simulink model "power_KundurTwoAreaSystem"  (R2021b)
settings: Solver=VariableStepAuto  StartTime=0.0  StopTime=20  MaxStep=1/60  RelTol=1e-4
PreLoadFcn:
  | Ts=50e-6;
  | Tctrl=2*Ts;
  | PSSMODEL=1;
model workspace (MAT data in the model file):
  LOL = 0
undefined symbols (not defined in the file or in its folder): D1, Delta
libraries: spsGenericPowerSystemStabilizerLib x8, spsThreePhaseVIMeasurementLib x6, spsLoadFlowBusLib x6, spsThreePhaseParallelRLCLoadLib x4, spsThreePhasePISectionLineLib x4, spsSynchronousMachinepuStandardLib x4, spsExcitationSystemLib x4, spsSteamTurbineandGovernorLib x4, spsThreePhaseSeriesRLCLoadLib x4, spsThreePhaseTransformerTwoWindingsLib x4, spsThreePhaseBreakerLib x2, spsDistributedParametersLineLib x2
(part 1 of 2)
settings Model: ARTEMISmethode_block_infos=$$__separator__$$  Creator=The MathWorks, Inc.  LastModifiedBy=Pavel
settings SolverCC: AlgebraicLoopSolver=TrustRegion
settings DataIOCC: SaveOutput=off  SignalLogging=off  DSMLogging=off  SaveTime=off  ReturnWorkspaceOutputs=off  TimeSaveName=t  SignalLoggingName=sigsOut
settings OptimizationCC: BlockReduction=off  BooleanDataType=off  OptimizeBlockIOStorage=off  BufferReuse=off  GlobalBufferReuse=off  ExpressionFolding=off  ExpressionDepthLimit=2147483647  LocalBlockOutputs=off  InitFltsAndDblsToZero=on  LifeSpan=inf  OptimizeDataStoreBuffers=off  BusAssignmentInplaceUpdate=off
settings DebuggingCC: SaveWithParameterizedLinksMsg=none  SignalResolutionControl=TryResolveAllWithWarning  MultiTaskDSMMsg=warning  MultiTaskCondExecSysMsg=none  FcnCallInpInsideContextMsg=warning  UnconnectedOutputMsg=none  StateNameClashWarn=warning  SFUnexpectedBacktrackingDiag=warning  SFNoUnconditionalDefaultTransitionDiag=warning  SFExecutionAtInitializationDiag=none  SFMachineParentedDataDiag=warning  ArithmeticOperatorsInVariantConditions=warning
settings HardwareCC: ProdBitPerPointer=32  ProdBitPerSizeT=32  ProdBitPerPtrDiffT=32  ProdLargestAtomicFloat=None  ProdIntDivRoundTo=Undefined  ProdEndianess=Unspecified  ProdWordSize=32  ProdHWDeviceType=32-bit Generic  TargetBitPerPointer=64  TargetBitPerSizeT=64  TargetBitPerPtrDiffT=64  TargetLongLongMode=on  TargetIntDivRoundTo=Zero  TargetEndianess=LittleEndian  TargetWordSize=64  TargetHWDeviceType=MATLAB Host  ProdEqTarget=off
settings ModelReferenceCC: PropagateSignalLabelsOutOfModel=off
settings SFSimCC: SimUseLocalCustomCode=off  CustomCodeUndefinedFunction=UseInterfaceOnly
settings RTWCC: RTWUseLocalCustomCode=off
settings CodeAppCC: StateflowObjectComments=on
settings GRTTargetCC: TargetFcnLib=ansi_tfl_tmw.mat  TargetLangStandard=C89/C90 (ANSI)  CombineOutputUpdateFcns=off  GRTInterface=on
settings ConfigComp: CovMetricSettings=dw  CovSaveCumulativeToWorkspaceVar=on  CovSaveSingleToWorkspaceVar=on  CovExternalEMLEnable=off  CovSFcnEnable=off
settings SimscapeCC: SimscapeNormalizeSystem=off  SimscapeNominalValues={1, 'bar'; 1, 'cm^3/s'; 1, 'bar*kg/s'; 1, 'kJ/kg'; 1, 'kW'; }

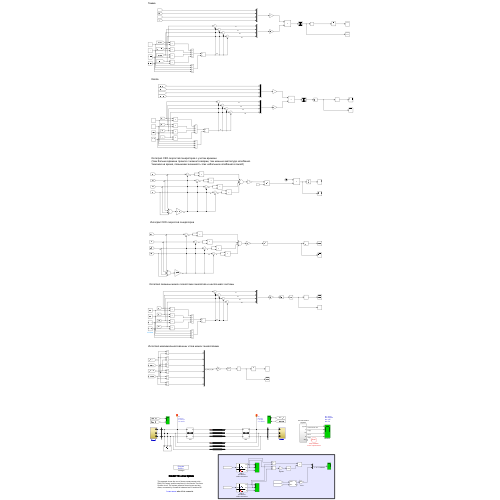
[thumbnail: Simulink's stored preview of the top-level diagram]
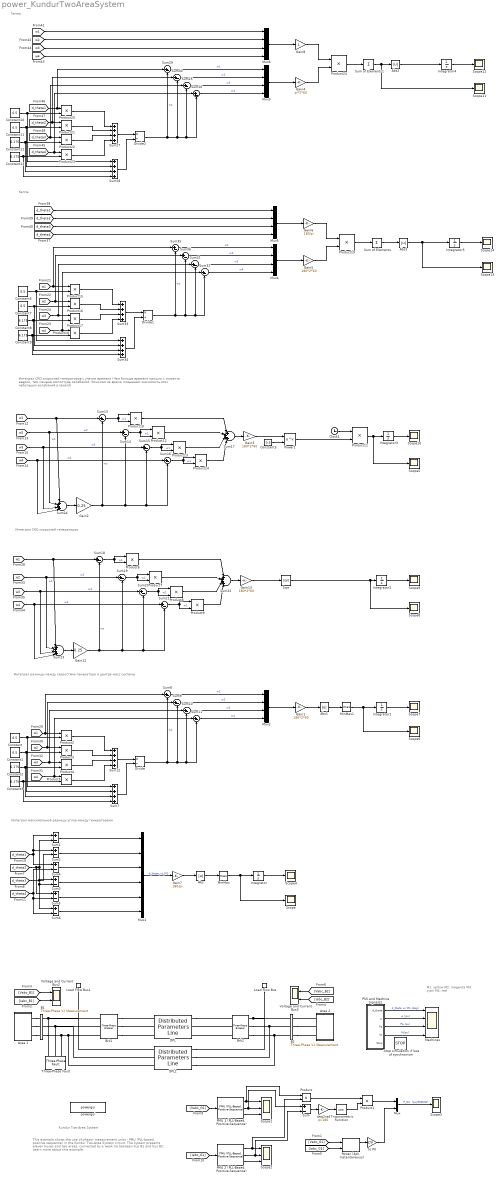
== system power_KundurTwoAreaSystem ==
  note: Интеграл максимальной разницы углов между генераторами
  note: This example shows the use of phasor measurement units - PMU (PLL-based, positive sequence) in the Kundur Two-Area System circuit. The system presents eleven buses and two areas, connected by a weak tie between bus B1 and bus B2.
      |
      | Learn more about this example.
  note: M1: yellow
      | M2: magenta
      | M3: cyan
      | M4: red
  note: Kundur Two-Area System
  note: Интеграл разницы между скоростями генератора и центра масс системы
  note: Интеграл СКО скоростей генераторов
  note: Интеграл СКО скоростей генераторов с учетом времени
      | (Чем больше времени прошло с момента аварии, тем меньше амплитуда колебаний. Умножая на время, повышаем значимость этих небольших колебаний в reward)
  note: Каппа
  note: Гамма
  " Brk2" : spsThreePhaseBreakerLib/Three-Phase Breaker  InitialState=closed  SwitchA=on  SwitchB=on  SwitchC=on  SwitchTimes=[2+12]*100  External=off  BreakerResistance=0.001  SnubberResistance=1e6  SnubberCapacitance=0  Measurements=None
      settings: AttributesFormatString=\n
  Abs{,1..3} (4 alike) : Abs  SaturateOnIntegerOverflow=on
  Area 1 : Subsystem
  Area 2 : Subsystem
  B1 : spsThreePhaseVIMeasurementLib/Three-Phase V-I Measurement  VoltageMeasurement=phase-to-ground  SetLabelV=on  LabelV=Vabc_B1  Vpu=on  VpuLL=off  CurrentMeasurement=yes  SetLabelI=on  LabelI=Iabc_B1  Ipu=off  Pbase=100e6  Vbase=230e3  OutputType=Complex  PhasorSimulation=off  PSBequivalent=0
  B2 : spsThreePhaseVIMeasurementLib/Three-Phase V-I Measurement  VoltageMeasurement=phase-to-ground  SetLabelV=on  LabelV=Vabc_B2  Vpu=off  VpuLL=off  CurrentMeasurement=yes  SetLabelI=on  LabelI=Iabc_B2  Ipu=off  Pbase=100e6  Vbase=500e3  OutputType=Complex  PhasorSimulation=off  PSBequivalent=0
  Brk1 : spsThreePhaseBreakerLib/Three-Phase Breaker  InitialState=closed  SwitchA=off  SwitchB=off  SwitchC=off  SwitchTimes=[2+12]  External=off  BreakerResistance=0.001  SnubberResistance=inf  SnubberCapacitance=0  Measurements=None
      settings: AttributesFormatString=\n
  Clock1 : Clock
  Constant{,1,6..7,10..11} (6 alike) : Constant  Value=6.5
  Constant{2..3,8..9,12..13} (6 alike) : Constant  Value=6.175
  Constant5 : Constant  Value=0.5
  DPL : spsDistributedParametersLineLib/Distributed Parameters Line  Phases=3  Length=220  Frequency=60  Resistance=[0.0001*529 1.61]  Inductance=[0.001*529/(377) 0.0061]  Capacitance=[0.00175/529/(377) 5.2489e-9]  x1=[-0.00125 4.24168847071057e-05 242154.913453712 -378268.611075755;-0.0012 3.78652229655789e-05 249241.699355128 -373637.156528352;-0.00115 3.33001078906322e-05 256239.930867557 -368872.950478352;-0.0011 2.87231614459144e-05 263147.121552666 -363977.68562548;-0.00105 2.41360097987035e-05 269960.817318493 -358953.101234027;-0.001 1.95402827421377e-05 276678.597291377 -353800.982514903;-0.00095 1.49376131161569e-05 283298.074676081 -348523.159991357;-0.0009 1.03296362273631e-05 289816.897603809 -343121.5088486;-0.00085 5.71798926800358e-06 296232.749967817 -337597.948267562;-0.0008 1.10431073428398e-06 302543.352246308 -331954.440743018;-0.00075 -3.50976015578118e-06 308746.462312342 -326192.991386318;-0.0007 -8.12258404477517e-06 314839.876230449 -320315.647212985;-0.00065 -1.27325220183347e-05 320821.429039679 -314324.496415418;-0.0006 -1.73379361874485e-05 326688.9955228 -308221.667620967;-0.00055 -2.19371902703915e-05 332440.49096138 -302009.329135645;-0.0005 -2.6528650174088e-05 338073.871876476 -295689.688173734;-0.00045 -3.11106845746969e-05 343587.136754673 -289264.990073576;-0.0004 -3.56816654972136e-05 348978.326759211 -282737.517499814;-0.00035 -4.02399688938816e-05 354245.526425954 -276109.589632373;-0.0003 -4.4783975221209e-05 359386.86434394 -269383.561342464;-0.00025 -4.93120700153845e-05 364400.513820286 -262561.822355911;-0.0002 -5.38226444658888e-05 369284.693529209 -255646.796404095;-0.00015 -5.83140959870971e-05 374037.668144913 -248640.940362808;-0.0001 -6.27848287876708e-05 378657.74895815 -241546.743379344;-5e-05 -6.72332544375335e-05 383143.294476206 -234366.72598811]  x2=[-0.00125 0.000104496170581926 -84178.9423133657 -331460.289661515;-0.0012 0.000103951893551609 -77916.4724740299 -332988.025993747;-0.00115 0.000103370682908492 -71626.3192830326 -334397.453265906;-0.0011 0.00010275274515395 -65310.7176018511 -335688.070715193;-0.00105 0.000102098299838323 -58971.9113336904 -336859.419791372;-0.001 0.000101407579482918 -52612.1526262346 -337911.084319696;-0.00095 0.000100680829497386 -46233.7010714696 -338842.690648764;-0.0009 9.9918308092537e-05 -39838.8229028612 -339653.907783284;-0.00085 9.91202861885959e-05 -33429.7901901726 -340344.447501671;-0.0008 9.8287047318945e-05 -27008.8800322094 -340914.064458451;-0.00075 9.7418887529387e-05 -20578.3737477767 -341362.556271432;-0.0007 9.65161152729613e-05 -14140.5560651377 -341689.763593607;-0.00065 9.5579051300352e-05 -7697.71431026073 -341895.570169774;-0.0006 9.46080285459267e-05 -1252.13759414292 -341979.902877835;-0.00055 9.36033920094462e-05 5193.88400049989 -341942.731754782;-0.0005 9.25654986334885e-05 11638.0602328886 -341784.070007336;-0.00045 9.14947171766277e-05 18078.1015178926 -341503.974007263;-0.0004 9.0391428082417e-05 24511.7197395083 -341102.543271336;-0.00035 8.92560233442181e-05 30936.629063816 -340579.920425984;-0.0003 8.80889063659281e-05 37350.5467511257 -339936.291156617;-0.00025 8.6890491818652e-05 43751.1939670238 -339171.884141649;-0.0002 8.5661205493372e-05 50136.2965920319 -338286.970971252;-0.00015 8.44014841496662e-05 56503.5860295907 -337281.866050863;-0.0001 8.31117753605297e-05 62850.8000120818 -336156.926489473;-5e-05 8.1792537353354e-05 69175.6834046 -334912.551972752]  x3=[-0.00125 -1.30073036814727e-07 581.32351976172 1802.01651045561;-0.0012 -1.28650380987693e-07 547.255027379994 1812.65326992482;-0.00115 -1.27182016292879e-07 512.992097892859 1822.64600231838;-0.0011 -1.25668464433268e-07 478.546904756015 1831.99115726607;-0.00105 -1.24110263166629e-07 443.931686182569 1840.68541447882;-0.001 -1.22507966114453e-07 409.158740794855 1848.72568492845;-0.00095 -1.20862142565252e-07 374.240423254795 1856.10911194515;-0.0009 -1.19173377272298e-07 339.189139874342 1862.83307223245;-0.00085 -1.17442270245856e-07 304.017344207581 1868.89517679929;-0.0008 -1.15669436540012e-07 268.737532626037 1874.29327180878;-0.00075 -1.13855506034138e-07 233.362239878777 1879.02543934347;-0.0007 -1.12001123209107e-07 197.904034638869 1883.08999808676;-0.00065 -1.10106946918306e-07 162.375515037798 1886.48550392028;-0.0006 -1.08173650153553e-07 126.789304189405 1889.21075043698;-0.00055 -1.06201919805981e-07 91.1580457049546 1891.26476936975;-0.0005 -1.04192456421996e-07 55.4943992009252 1892.64683093545;-0.00045 -1.02145973954368e-07 19.811035801103 1893.35644409418;-0.0004 -1.00063199508575e-07 -15.8793663654067 1893.39335672376;-0.00035 -9.79448730844584e-08 -51.5641266686583 1892.75755570931;-0.0003 -9.57917473133114e-08 -87.2305664832333 1891.4492669479;-0.00025 -9.36045871904677e-08 -122.866013692895 1889.46895526831;-0.0002 -9.13841698035045e-08 -158.457807192933 1886.81732426584;-0.00015 -8.91312840561466e-08 -193.993301388591 1883.49531605237;-0.0001 -8.68467303879727e-08 -229.459870687988 1879.50411092158;-5e-05 -8.45313204900229e-08 -264.844913987929 1874.84512692967]  x4=[-0.00125 2.86918544594886e-07 -451.193099671548 -3595.35316184637;-0.0012 2.82321210867361e-07 -383.346048401822 -3603.21848238076;-0.00115 2.7762356975792e-07 -315.362796106445 -3609.80359654552;-0.0011 2.72827290316081e-07 -247.26749691125 -3615.10616468092;-0.00105 2.67934076637092e-07 -179.084344751795 -3619.12430280977;-0.001 2.62945667256474e-07 -110.837564777381 -3621.85658330673;-0.00095 2.57863834532326e-07 -42.551404743968 -3623.30203540552;-0.0009 2.52690384015618e-07 25.7498736009369 -3623.46014554392;-0.00085 2.47427153808685e-07 94.0420031383625 -3622.33085754614;-0.0008 2.42076013912157e-07 162.300719999866 -3619.91457264283;-0.00075 2.36638865560559e-07 230.501772188366 -3616.21214932852;-0.0007 2.31117640546812e-07 298.62092819477 -3611.22490305656;-0.00065 2.25514300535872e-07 366.633985607305 -3604.95460577182;-0.0006 2.19830836367765e-07 434.516779710524 -3597.40348528107;-0.00055 2.14069267350247e-07 502.245192070916 -3588.57422446146;-0.0005 2.08231640541355e-07 569.795159106064 -3578.46996030732;-0.00045 2.02320030022099e-07 637.142680634329 -3567.09428281559;-0.0004 1.96336536159546e-07 704.263828401995 -3554.45123371032;-0.00035 1.90283284860576e-07 771.134754584864 -3540.54530500664;-0.0003 1.8416242681655e-07 837.731700261279 -3525.38143741482;-0.00025 1.77976136739188e-07 904.03100385355 -3508.96501858481;-0.0002 1.71726612587897e-07 970.009109534801 -3491.30188119205;-0.00015 1.65416074788851e-07 1035.64257559825 -3472.39830086514;-0.0001 1.59046765446079e-07 1100.90808278592 -3452.26099395617;-5e-05 1.52620947544865e-07 1165.78244257388 -3430.8971151544]  x5=0.00124486354111605  V1=[1.852e-10 2.282e+05 2.282e+05;377 377 377;1.887 0.4815 -1.089]  V2=[4.602e-11 2.307e+05 2.307e+05;377 377 377;0.7797 0.0189 -1.552]  I1=[2.265e-13 336.1 336.1;377 377 377;-2.48 -2.709 2.004]  I2=[2.156e-13 1427 1427;377 377 377;2.209 0.1789 -1.392]  nHarmo=1  Measurements=None  Decoupling=off  VsMag0=0  VrMag0=0  VsAngle0=0  VrAngle0=0  IsMag0=0  IrMag0=0  IsAngle0=0  IrAngle0=0
      settings: SourceProductBaseCode=PS
  DPL2 : spsDistributedParametersLineLib/Distributed Parameters Line  Phases=3  Length=220  Frequency=60  Resistance=[0.0001*529 1.61]  Inductance=[0.001*529/(377) 0.0061]  Capacitance=[0.00175/529/(377) 5.2489e-9]  x1=[-0.00125 4.24158242213737e-05 242154.924794119 -378271.378614112;-0.0012 3.78640919415657e-05 249241.762857399 -373639.923361119;-0.00115 3.32989067301852e-05 256240.046509131 -368875.715622486;-0.0011 2.87218905758001e-05 263147.289292455 -363980.448098539;-0.00105 2.41346696704561e-05 269961.037096901 -358955.860054517;-0.001 1.95388738318982e-05 276678.869030317 -353803.736702629;-0.00095 1.49361359245046e-05 283298.398279006 -348525.908567769;-0.0009 1.03280912791371e-05 289817.272955745 -343124.250837142;-0.00085 5.71637711211663e-06 296233.176935402 -337600.682694019;-0.0008 1.10263194352739e-06 302543.830677843 -331957.16663586;-0.00075 -3.51150498494106e-06 308746.992037843 -326195.707777049;-0.0007 -8.12439429240883e-06 314840.457061706 -320318.353136484;-0.00065 -1.27343970412698e-05 320822.060770326 -314327.190910284;-0.0006 -1.73398753194983e-05 326689.677928386 -308224.349729859;-0.00055 -2.19391928225916e-05 332441.223799449 -302011.997905621;-0.0005 -2.65307154349411e-05 338074.654886655 -295692.342656594;-0.00045 -3.11128118104258e-05 343587.969658762 -289267.629326194;-0.0004 -3.56838539520215e-05 348979.209261284 -282740.140584477;-0.00035 -4.02422177902209e-05 354246.458212461 -276112.195617111;-0.0003 -4.47862837600576e-05 359387.845083821 -269386.149301382;-0.00025 -4.93144373765294e-05 364401.543165091 -262564.391369521;-0.0002 -5.38250698082179e-05 369285.771113215 -255649.345559638;-0.00015 -5.8316578448898e-05 374038.79358526 -248643.468754582;-0.0001 -6.27873674869364e-05 378658.921854975 -241549.250109023;-5e-05 -6.72358484722762e-05 383144.514412783 -234369.210165065]  x2=[-0.00125 0.000104493504401818 -84178.6934931397 -331457.464505496;-0.0012 0.00010394919839188 -77916.2769478754 -332985.196649946;-0.00115 0.00010336795972672 -71626.1771204191 -334394.620739574;-0.0011 0.000102749994917668 -65310.6288532885 -335685.236012713;-0.00105 0.000102095523524678 -58971.8760307105 -336856.583919902;-0.001 0.00010140477807832 -52612.1707813803 -337908.248286806;-0.00095 0.000100678003997161 -46233.7726782906 -338839.855462084;-0.0009 9.99154595005715e-05 -39838.9479359159 -339651.074450143;-0.00085 9.91174155169812e-05 -33429.9686050373 -340341.617028737;-0.0008 9.8284155587617e-05 -27009.1117654942 -340911.237851378;-0.00075 9.74159757657642e-05 -20578.6587171479 -341359.7345345;-0.0007 9.65131845115794e-05 -14140.894169347 -341686.947729366;-0.00065 9.55761025824965e-05 -7698.10542918133 -341892.761178687;-0.0006 9.4605062919263e-05 -1252.58158881211 -341977.101757924;-0.00055 9.36004105276475e-05 5193.3872878313 -341939.93950127;-0.0005 9.25625023558609e-05 11637.5109787003 -341781.287612299;-0.00045 9.14917071677345e-05 18077.4999173319 -341501.202459272;-0.0004 9.03884054117e-05 24511.0660063211 -341099.783555109;-0.00035 8.92529890856178e-05 30935.9234302705 -340577.173522035;-0.0003 8.80858615975021e-05 37349.7894679302 -339933.558040908;-0.00025 8.6887437622192e-05 43750.3853032374 -339169.165785242;-0.0002 8.56581429540196e-05 50135.436834969 -338284.268339967;-0.00015 8.43984143555269e-05 56502.6754847189 -337279.180104931;-0.0001 8.31086994022867e-05 62849.8390029132 -336154.258183199;-5e-05 8.17894563238808e-05 69174.6722725767 -334909.902254172]  x3=[-0.00125 -1.3007666837781e-07 581.370317473745 1802.01238818334;-0.0012 -1.28654069730555e-07 547.301894480357 1812.6500304473;-0.00115 -1.27185760904926e-07 513.039017729903 1822.6436467866;-0.0011 -1.25672263584058e-07 478.593860659345 1831.98968651693;-0.00105 -1.24114115506341e-07 443.978661468976 1840.68482903487;-0.001 -1.22511870274369e-07 409.205718774244 1848.72598499769;-0.00095 -1.20866097158243e-07 374.287387236113 1856.11029742098;-0.0009 -1.19177380893315e-07 339.23607317151 1862.83514269367;-0.00085 -1.17446321472433e-07 304.064230145423 1868.89813151028;-0.0008 -1.15673533932766e-07 268.784354546202 1874.29710971974;-0.00075 -1.13859648137287e-07 233.408981145659 1879.0301590908;-0.0007 -1.1200530855098e-07 197.95067864552 1883.09559799356;-0.00065 -1.10111174011871e-07 162.422045211823 1886.49198199694;-0.0006 -1.08177917496943e-07 126.835703998855 1889.21810438187;-0.00055 -1.06206225883031e-07 91.2042986641984 1891.27299657004;-0.0005 -1.04196799702776e-07 55.5404888765067 1892.65592846806;-0.00045 -1.02150352895732e-07 19.85694581758 1893.36640872679;-0.0004 -1.00067612554704e-07 -15.8336523196446 1893.40418491599;-0.00035 -9.79493186674205e-08 -51.5186248355938 1892.76924361396;-0.0003 -9.57962238536111e-08 -87.185293029451 1891.46181041232;-0.00025 -9.36090930976116e-08 -122.820984703838 1889.48234983585;-0.0002 -9.13887034765653e-08 -158.413038667186 1886.83156517748;-0.00015 -8.91358438843318e-08 -193.948809232198 1883.51039824838;-0.0001 -8.68513147511971e-08 -229.4156707088 1879.52002904333;-5e-05 -8.45359277594841e-08 -264.801021889989 1874.86187532152]  x4=[-0.00125 2.86921266557822e-07 -451.239240117452 -3595.34899258331;-0.0012 2.82323919730767e-07 -383.392259238491 -3603.2151835324;-0.00115 2.77626264559351e-07 -315.409060915391 -3609.80116928392;-0.0011 2.72829970098087e-07 -247.313799254805 -3615.10460986848;-0.00105 2.67936740447559e-07 -179.130668178958 -3619.1236209989;-0.001 2.62948314148962e-07 -110.883892829658 -3621.85677473967;-0.00095 2.57866463566408e-07 -42.5977209612231 -3623.30310001427;-0.0009 2.5269299425721e-07 25.7035856746353 -3623.46208295022;-0.00085 2.4742974433038e-07 93.9957599488946 -3622.33366706165;-0.0008 2.42078583793556e-07 162.254537977216 -3619.91825326933;-0.00075 2.36641413888595e-07 230.455667740787 -3616.2166997583;-0.0007 2.31120166416076e-07 298.574917702953 -3611.23032167288;-0.00065 2.25516803048935e-07 366.588085418558 -3604.96089064947;-0.0006 2.19833314635496e-07 434.471006132967 -3597.41063418706;-0.00055 2.14071720492129e-07 502.199561367681 -3588.58223485583;-0.0005 2.08234067685799e-07 569.749687489525 -3578.478829344;-0.00045 2.02322430306751e-07 637.097384260333 -3567.10400734346;-0.0004 1.96338908731597e-07 704.218723364128 -3554.46181027429;-0.00035 1.90285628877062e-07 771.089856908732 -3540.55672984893;-0.0003 1.84164741444655e-07 837.687025898813 -3525.39370647622;-0.00025 1.77978421156534e-07 903.986568677336 -3508.97812750619;-0.0002 1.71728865982841e-07 969.964929332448 -3491.31582531586;-0.00015 1.65418296360772e-07 1035.59866606677 -3472.41307523712;-0.0001 1.59048954405665e-07 1100.86445952616 -3452.27659332704;-5e-05 1.52623103114388e-07 1165.73912108498 -3430.91353398178]  x5=0.00124486354111605  V1=[5.683e-11 2.282e+05 2.282e+05;377 377 377;0.4068 0.4815 -1.089]  V2=[7.166e-11 2.307e+05 2.307e+05;377 377 377;-0.05108 0.0189 -1.552]  I1=[2.676e-13 336.1 336.1;377 377 377;-1.905 -2.709 2.004]  I2=[9.643e-14 1427 1427;377 377 377;-2.04 0.1789 -1.392]  nHarmo=1  Measurements=None  Decoupling=off  VsMag0=0  VrMag0=0  VsAngle0=0  VrAngle0=0  IsMag0=0  IrMag0=0  IsAngle0=0  IrAngle0=0
      settings: SourceProductBaseCode=PS
  Divide : Product  Inputs=*/
  Divide1 : Product  Inputs=*/
  Divide2 : Product  Inputs=*/
  Gain{1,3,5,13} (4 alike) : Gain  Gain=180*2*60
  Gain12 : Gain  Gain=0.25
  Gain2 : Gain  Gain=0.25
  Gain4 : Gain  Gain=pi*2*60
  Gain6 : Gain  Gain=180/pi
  Gain7 : Gain  Gain=180/pi
  Gain8 : Gain
  Integrator{,1..5} (6 alike) : Integrator
  Load Flow Bus : spsLoadFlowBusLib/Load Flow Bus  LConnTagsString=a  Phases=single  Connectors=on one side  ID=B2  Vbase=230e3  Vref=1  Vangle=0  VLF=1.003  VLFb=1  VLFc=1  angleLF=-11.54  angleLFb=0  angleLFc=0
      settings: AttributesFormatString=%<ID>\n%<Vbase>V\n%<VLF>pu\n%<angleLF>deg.  SourceProductBaseCode=PS
  Load Flow Bus1 : spsLoadFlowBusLib/Load Flow Bus  LConnTagsString=a  Phases=single  Connectors=on one side  ID=B1  Vbase=230e3  Vref=1  Vangle=0  VLF=0.9914  VLFb=1  VLFc=1  angleLF=15.04  angleLFb=0  angleLFc=0
      settings: AttributesFormatString=%<ID>\n%<Vbase>V\n%<VLF>pu\n%<angleLF>deg.  SourceProductBaseCode=PS
  Machines : Scope  NumInputPorts=4
  MinMax : MinMax  Function=max  InputSameDT=on  SaturateOnIntegerOverflow=on
  MinMax1 : MinMax  Function=max  InputSameDT=on  SaturateOnIntegerOverflow=on
  Mux : Mux  Inputs=2
  Mux1 : Mux  Inputs=6
  Mux{2..6} (5 alike) : Mux
  "PMU 1 (PLL-Based, Positive-Sequence)" : spsPMUPLLBasedPositiveSequenceLib/PMU (PLL-Based, Positive-Sequence)  nominalFrequency=60  samplingRate=64  reportingFactor=1
      settings: SourceProductBaseCode=PS
  "PMU 2 (PLL-Based, Positive-Sequence)" : spsPMUPLLBasedPositiveSequenceLib/PMU (PLL-Based, Positive-Sequence)  nominalFrequency=60  samplingRate=64  reportingFactor=1
      settings: SourceProductBaseCode=PS
  PSS and Machine Signals2 : Subsystem
  "Power (3ph, Instantaneous)" : spsPower3phInstantaneousLib/Power (3ph, Instantaneous)
  Power1 : Math  Operator=pow  SaturateOnIntegerOverflow=on
  Product{,1..24} (25 alike) : Product
  Scope{,3..14} (13 alike) : Scope
  Scope1 : Scope  NumInputPorts=3
  Scope2 : Scope  NumInputPorts=3
  Sqrt : Sqrt  SaturateOnIntegerOverflow=on
  Stop simulation if loss of synchronism : Stop
  Sum : Sum  Inputs=+-
  Sum of Elements : Sum  Inputs=+
  Sum of Elements1 : Sum  Inputs=+
  Sum{1..6} (6 alike) : Sum  Inputs=+-  InputSameDT=on  SaturateOnIntegerOverflow=on  OutDataTypeStr=Inherit: Same as first input
  Sum{8..11,13..16,18..21,25..26,29..32,35..36} (20 alike) : Sum  Inputs=|+-
  Sum{7,12,27..28,33..34} (6 alike) : Sum  Inputs=++++  InputSameDT=on  SaturateOnIntegerOverflow=on  OutDataTypeStr=Inherit: Same as first input
  Sum{17,22..24} (4 alike) : Sum  Inputs=|++++|
  Three-Phase Fault : spsThreePhaseFaultLib/Three-Phase Fault  InitialStates=0  FaultA=on  FaultB=on  FaultC=on  GroundFault=on  SwitchTimes=[20 20.25]  External=off  SwitchStatus=NaN  FaultResistance=0.001  GroundResistance=0.001  SnubberResistance=1e6  SnubberCapacitance=inf  Measurements=None
  Trigonometric Function : Trigonometry  Operator=cos
  Voltage and Current Bus2 : Scope  NumInputPorts=2
  Voltage and Current Bus3 : Scope  NumInputPorts=2
  deg2rad : Gain  Gain=pi/180
  powergui : spspowerguiLib/powergui  Priority=2  SimulationMode=Discrete  SampleTime=Ts  frequency=60  Iterations=50  frequencyindice=60  Pbase=100e6  ErrMax=1e-4  UnitsV=kV  UnitsW=MW  buscounter=0  FunctionMessages=off  echomessages=off  EnableUseOfTLC=off  CurrentSourceSwitches=off  DisableSnubberDevices=off  DisableRonSwitches=off  DisableVfSwitches=off  DisplayEquations=off  AutomaticDiscreteSolvers=off  SolverType=Tustin  Interpol=off  ExternalGateDelay=off  methode=off  Ts=0  x0status=blocks  SPID=off  SwTol=0  HookPort=off  NonlinearTolerance=1e-4  nMaxIteration=100  ContinueOnMaxIteration=off  RestoreLinks=warning  ResistiveCurrentMeasurement=off  Frange=logspace(0,3,50)  Ylog=off  Xlog=off  ShowGrid=off  save=off  variable=ZData  structure=0  ZoomFFT=on  StartTime=0.0  cycles=1  DisplayStyle=1  fundamental=60  FreqAxis=off  MaxFrequency=1000  frequencyindicesteady=1  RmsSteady=1  display=off
  to PU : Gain  Gain=2/3
  wires:
  [Iabc_B1] -> Voltage and Current Bus2/2
  [Vabc_B1] -> Voltage and Current Bus2/1
  [Iabc_B2] -> Voltage and Current Bus3/2
  [Vabc_B2] -> Voltage and Current Bus3/1
  PSS and Machine Signals2/1(d_theta) -> Machines/1  "d_theta vs M1 (deg)"
  PSS and Machine Signals2/2(w) -> Machines/2  "w (pu)"
  PSS and Machine Signals2/3(Pa) -> Machines/3  "Pa (pu)"
  PSS and Machine Signals2/4(Vt) -> Machines/4  "Vt(pu)"
  [Iabc_G1] -> "PMU 2 (PLL-Based, Positive-Sequence)"/1
  "PMU 2 (PLL-Based, Positive-Sequence)"/3 -> Scope2/3
  [Vabc_G1] -> "PMU 1 (PLL-Based, Positive-Sequence)"/1
  "PMU 1 (PLL-Based, Positive-Sequence)"/3 -> Scope1/3
  Product/1 -> Product1/1
  [Iabc_G1] -> "Power (3ph, Instantaneous)"/2
  "Power (3ph, Instantaneous)"/1 -> to PU/1
  "PMU 2 (PLL-Based, Positive-Sequence)"/1 -> Product/2, Scope2/1
  [Vabc_G1] -> "Power (3ph, Instantaneous)"/1
  "PMU 2 (PLL-Based, Positive-Sequence)"/2 -> Sum/2, Scope2/2
  deg2rad/1 -> Trigonometric Function/1
  "PMU 1 (PLL-Based, Positive-Sequence)"/1 -> Scope1/1, Product/1
  Trigonometric Function/1 -> Product1/2
  Product1/1 -> Mux/1
  Sum/1 -> deg2rad/1
  to PU/1 -> Mux/2
  "PMU 1 (PLL-Based, Positive-Sequence)"/2 -> Sum/1, Scope1/2
  Mux/1 -> Scope3/1  "P_G1  (pu/900MW)"
  Sum4/1 -> Mux1/3
  Sum2/1 -> Mux1/2
  Sum1/1 -> Mux1/1
  Gain7/1 -> Abs/1
  Abs/1 -> MinMax/1
  Sum5/1 -> Mux1/5
  Sum3/1 -> Mux1/4
  [d_theta1] -> Sum4/1, Sum2/1, Sum1/1
  [d_theta2] -> Sum5/1, Sum1/2, Sum3/1
  [d_theta3] -> Sum6/1, Sum3/2, Sum2/2
  [d_theta4] -> Sum6/2, Sum5/2, Sum4/2
  Mux1/1 -> Gain7/1  "d_theta_vs_M1"
  MinMax/1 -> Integrator/1, Scope/1
  Integrator/1 -> Scope4/1
  Product2/1 -> Sum12/1
  [w1] -> Product2/1, Sum8/1
  [w3] -> Product4/1, Sum10/1
  Sum9/1 -> Mux2/2  "w2"
  Divide/1 -> Sum9/2, Sum10/2, Sum11/2, Sum8/2  "ws"
  [w4] -> Product5/1, Sum11/1
  Sum11/1 -> Mux2/4  "w4"
  Sum8/1 -> Mux2/1  "w1"
  Sum10/1 -> Mux2/3  "w3"
  [w2] -> Product3/1, Sum9/1
  Constant/1 -> Sum7/1, Product2/2
  Constant1/1 -> Sum7/2, Product3/2
  Constant2/1 -> Sum7/3, Product4/2
  Constant3/1 -> Sum7/4, Product5/2
  Product3/1 -> Sum12/2
  Product4/1 -> Sum12/3
  Product5/1 -> Sum12/4
  Sum12/1 -> Divide/1
  Sum7/1 -> Divide/2
  Gain1/1 -> Abs1/1
  Abs1/1 -> MinMax1/1
  MinMax1/1 -> Integrator1/1, Scope6/1
  Integrator1/1 -> Scope7/1
  Mux2/1 -> Gain1/1
  Sqrt/1 -> Scope8/1, Integrator2/1
  Sum23/1 -> Gain12/1
  Product9/1 -> Sum22/4
  Product8/1 -> Sum22/3
  Gain12/1 -> Sum18/2, Sum19/2, Sum20/2, Sum21/2  "ws"
  Product7/1 -> Sum22/2
  Sum21/1 -> Product9/1, Product9/2  "w1"
  Sum22/1 -> Gain13/1
  Sum19/1 -> Product7/1, Product7/2  "w1"
  Product6/1 -> Sum22/1
  [w2] -> Sum23/2, Sum19/1  "w2"
  [w4] -> Sum23/4, Sum21/1  "w4"
  [w1] -> Sum23/1, Sum18/1  "w1"
  Integrator2/1 -> Scope9/1
  Sum18/1 -> Product6/2, Product6/1  "w1"
  Sum20/1 -> Product8/2, Product8/1  "w1"
  [w3] -> Sum23/3, Sum20/1  "w3"
  Gain13/1 -> Sqrt/1
  Integrator3/1 -> Scope10/1
  Clock1/1 -> Product11/1
  Product11/1 -> Scope5/1, Integrator3/1
  Gain3/1 -> Power1/1
  [w3] -> Sum15/1, Sum24/3  "w3"
  Sum15/1 -> Product13/1, Product13/2  "w1"
  Sum13/1 -> Product10/1, Product10/2  "w1"
  [w1] -> Sum13/1, Sum24/1  "w1"
  Constant5/1 -> Power1/2
  [w4] -> Sum16/1, Sum24/4  "w4"
  [w2] -> Sum14/1, Sum24/2  "w2"
  Product10/1 -> Sum17/1
  Sum14/1 -> Product12/2, Product12/1  "w1"
  Sum17/1 -> Gain3/1
  Sum16/1 -> Product14/2, Product14/1  "w1"
  Product12/1 -> Sum17/2
  Gain2/1 -> Sum16/2, Sum15/2, Sum14/2, Sum13/2  "ws"
  Product13/1 -> Sum17/3
  Product14/1 -> Sum17/4
  Sum24/1 -> Gain2/1
  Power1/1 -> Product11/2
  Constant9/1 -> Sum34/4, Product18/2
  Constant6/1 -> Sum34/1, Product15/2
  Sum36/1 -> Mux4/2  "w2"
  [w1] -> Product15/1, Sum35/1
  [w3] -> Product17/1, Sum31/1
  Sum31/1 -> Mux4/3  "w3"
  [w2] -> Product16/1, Sum36/1
  Sum32/1 -> Mux4/4  "w4"
  [w4] -> Product18/1, Sum32/1
  Divide1/1 -> Sum36/2, Sum31/2, Sum32/2, Sum35/2  "ws"
  Product17/1 -> Sum33/3
  Product18/1 -> Sum33/4
  Sum35/1 -> Mux4/1  "w1"
  Sum34/1 -> Divide1/2
  Mux4/1 -> Gain5/1
  Integrator5/1 -> Scope14/1
  Product16/1 -> Sum33/2
  Abs3/1 -> Scope13/1, Integrator5/1
  Constant7/1 -> Sum34/2, Product16/2
  Sum33/1 -> Divide1/1
  Constant8/1 -> Sum34/3, Product17/2
  Product15/1 -> Sum33/1
  [d_theta3] -> Mux5/3
  [d_theta4] -> Mux5/4
  [d_theta2] -> Mux5/2
  [d_theta1] -> Mux5/1
  Mux5/1 -> Gain6/1
  Gain6/1 -> Product19/1
  Gain5/1 -> Product19/2
  Product19/1 -> Sum of Elements/1
  Sum of Elements/1 -> Abs3/1
  Sum of Elements1/1 -> Scope11/1, Abs2/1
  Product24/1 -> Sum of Elements1/1
  Gain4/1 -> Product24/2
  Gain8/1 -> Product24/1
  Mux6/1 -> Gain8/1
  [w1] -> Mux6/1
  [w2] -> Mux6/2
  [w4] -> Mux6/4
  [w3] -> Mux6/3
  Product20/1 -> Sum27/1
  Constant12/1 -> Product22/2, Sum28/3
  Sum27/1 -> Divide2/1
  Constant11/1 -> Product21/2, Sum28/2
  Abs2/1 -> Integrator4/1
  Product21/1 -> Sum27/2
  Integrator4/1 -> Scope12/1
  Mux3/1 -> Gain4/1
  Sum28/1 -> Divide2/2
  Sum29/1 -> Mux3/1  "w1"
  Product23/1 -> Sum27/4
  Product22/1 -> Sum27/3
  Divide2/1 -> Sum29/2, Sum26/2, Sum25/2, Sum30/2  "ws"
  [d_theta4] -> Sum26/1, Product23/1
  Sum26/1 -> Mux3/4  "w4"
  [d_theta2] -> Product21/1, Sum30/1
  Sum25/1 -> Mux3/3  "w3"
  [d_theta3] -> Product22/1, Sum25/1
  [d_theta1] -> Product20/1, Sum29/1
  Sum30/1 -> Mux3/2  "w2"
  Constant10/1 -> Product20/2, Sum28/1
  Constant13/1 -> Product23/2, Sum28/4
  Sum6/1 -> Mux1/6
  connections:
  " Brk2"/RConn1 -- DPL2/RConn1 -- B2/LConn1 -- Load Flow Bus/LConn1
  " Brk2"/RConn2 -- DPL2/RConn2 -- B2/LConn2
  " Brk2"/RConn3 -- DPL2/RConn3 -- B2/LConn3
  B2/RConn3 -- Area 2/LConn3
  B2/RConn2 -- Area 2/LConn2
  Area 2/LConn1 -- B2/RConn1
  Area 1/RConn3 -- B1/LConn3
  Area 1/RConn2 -- B1/LConn2
  Area 1/RConn1 -- B1/LConn1
  " Brk2"/LConn3 -- DPL/RConn3
  " Brk2"/LConn2 -- DPL/RConn2
  DPL/RConn1 -- " Brk2"/LConn1
  Brk1/RConn3 -- DPL/LConn3
  Brk1/RConn2 -- DPL/LConn2
  Brk1/RConn1 -- DPL/LConn1
  DPL2/LConn3 -- B1/RConn3 -- Three-Phase Fault/LConn3 -- Brk1/LConn3
  DPL2/LConn2 -- Brk1/LConn2 -- Three-Phase Fault/LConn2 -- B1/RConn2
  DPL2/LConn1 -- Brk1/LConn1 -- Load Flow Bus1/LConn1 -- Three-Phase Fault/LConn1 -- B1/RConn1

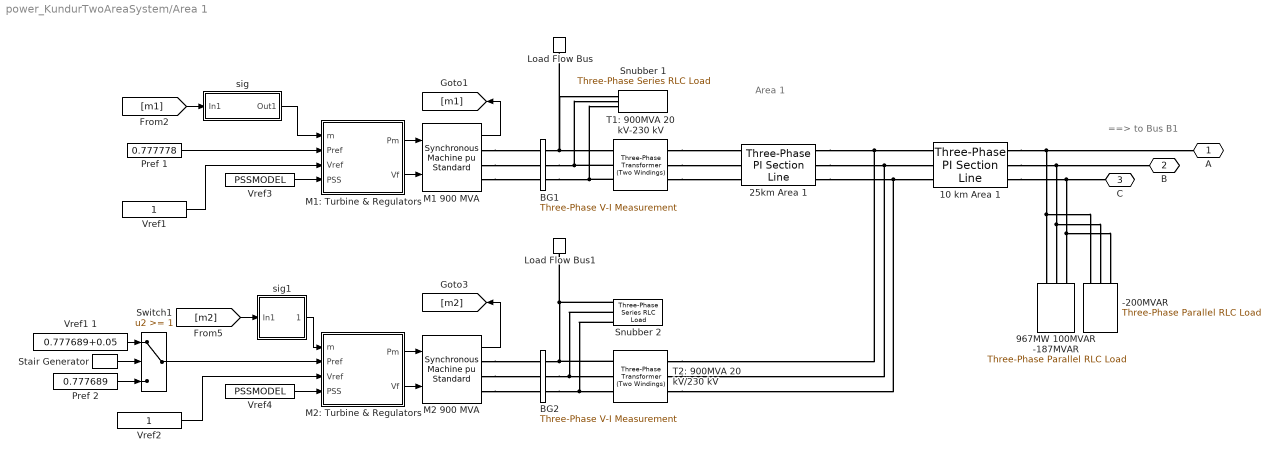
== system power_KundurTwoAreaSystem/Area 1 ==
  note: Area 1
  note: ==> to Bus B1
  -200MVAR : spsThreePhaseParallelRLCLoadLib/Three-Phase Parallel RLC Load  LConnTagsString=A|B|C  Configuration=Y (grounded)  NominalVoltage=230e3  Vabc=[1e3 1e3 1e3]  Vabcp=[1e3 1e3 1e3]  NominalFrequency=60  UnbalancedPower=off  ActivePower=0  InductivePower=0  CapacitivePower=200e6  Pabc=[10e3 9e3 11e3]  QLabc=[100 90 110]  QCabc=[100 90 110]  Pabcp=[10e3 9e3 11e3]  QLabcp=[100 90 110]  QCabcp=[100 90 110]  Measurements=None  LoadType=constant Z
  10 km Area 1 : spsThreePhasePISectionLineLib/Three-Phase PI Section Line  LConnTagsString=a|b|c  RConnTagsString=A|B|C  Length=10  Frequency=60  Resistances=[0.0001*529 1.61]  Inductances=[0.001*529/(377) 0.0061]  Capacitances=[0.00175/529/(377) 5.2489e-9]
  25km Area 1 : spsThreePhasePISectionLineLib/Three-Phase PI Section Line  LConnTagsString=a|b|c  RConnTagsString=A|B|C  Length=25  Frequency=60  Resistances=[0.0001*529 1.61]  Inductances=[0.001*529/(377) 0.0061]  Capacitances=[0.00175/529/(377) 5.2489e-9]
  967MW 100MVAR -187MVAR : spsThreePhaseParallelRLCLoadLib/Three-Phase Parallel RLC Load  LConnTagsString=A|B|C  Configuration=Y (grounded)  NominalVoltage=230e3  Vabc=[1e3 1e3 1e3]  Vabcp=[1e3 1e3 1e3]  NominalFrequency=60  UnbalancedPower=off  ActivePower=167e6  InductivePower=100e6  CapacitivePower=187e6  Pabc=[10e3 9e3 11e3]  QLabc=[100 90 110]  QCabc=[100 90 110]  Pabcp=[10e3 9e3 11e3]  QLabcp=[100 90 110]  QCabcp=[100 90 110]  Measurements=None  LoadType=constant Z
  BG1 : spsThreePhaseVIMeasurementLib/Three-Phase V-I Measurement  VoltageMeasurement=phase-to-ground  SetLabelV=on  LabelV=Vabc_G1  Vpu=on  VpuLL=off  CurrentMeasurement=yes  SetLabelI=on  LabelI=Iabc_G1  Ipu=on  Pbase=900e6  Vbase=20e3  OutputType=Complex  PhasorSimulation=off  PSBequivalent=0
  BG2 : spsThreePhaseVIMeasurementLib/Three-Phase V-I Measurement  VoltageMeasurement=no  SetLabelV=on  LabelV=Vabc_G2  Vpu=on  VpuLL=off  CurrentMeasurement=no  SetLabelI=on  LabelI=Iabc_G2  Ipu=on  Pbase=900e6  Vbase=20e3  OutputType=Complex  PhasorSimulation=off  PSBequivalent=0
  Load Flow Bus : spsLoadFlowBusLib/Load Flow Bus  LConnTagsString=a  Phases=single  Connectors=on one side  ID=M1_Area1  Vbase=20e3  Vref=1  Vangle=0  VLF=1  VLFb=1  VLFc=1  angleLF=10.19  angleLFb=0  angleLFc=0
      settings: AttributesFormatString=%<ID>\n%<Vbase>V\n%<VLF>pu\n%<angleLF>deg.  SourceProductBaseCode=PS
  Load Flow Bus1 : spsLoadFlowBusLib/Load Flow Bus  LConnTagsString=a  Phases=single  Connectors=on one side  ID=M2_Area1  Vbase=20e3  Vref=1  Vangle=0  VLF=1  VLFb=1  VLFc=1  angleLF=0  angleLFb=0  angleLFc=0
      settings: AttributesFormatString=%<ID>\n%<Vbase>V\n%<VLF>pu\n%<angleLF>deg.  SourceProductBaseCode=PS
  M1 900 MVA : spsSynchronousMachinepuStandardLib/Synchronous Machine pu Standard  PresetModel=No  MechanicalLoad=Mechanical power Pm  ShowDetailedParameters=on  RotorType=Round  Units=per unit standard parameters  MeasurementBus=off  NominalParameters="[900E6  20000   60 ]"  Reactances1=[1.8 .3 .25 1.7 .55 .25 .2]  Reactances2=[ 1.305, 0.296, 0.252, 0.474, 0.243, 0.18 ]  dAxisTimeConstants=Open-circuit  qAxisTimeConstants=Open-circuit  TimeConstants1=[]  TimeConstants2=[8 .03 .4 .05]  TimeConstants3=[]  TimeConstants4=[]  TimeConstants5=[ 1.01, 0.053, 0.1 ]  TimeConstants6=[]  TimeConstants7=[]  TimeConstants8=[]  StatorResistance=0.0025  Mechanical="[ 6.5 0  4]"  PolePairs=4  InitialConditions=[0 -31.4247 0.784453 0.784453 0.784453 2.7401 -117.26 122.74 1.83395]  SetSaturation=off  Saturation=[0.6404,0.7127,0.8441,0.9214,0.9956,1.082,1.19,1.316,1.457;0.7,0.7698,0.8872,0.9466,0.9969,1.046,1.1,1.151,1.201]  LoadFlowParameters=[1 700000000 0 0 0]  TsPowergui=0  TsBlock=-1  IterativeModel=Trapezoidal non iterative  IterativeDiscreteModel=Trapezoidal non iterative  BusType=PV  Pref=700000000  Qref=0  Qmin=-inf  Qmax=inf  PLF=0  QLF=0
      settings: SourceProductBaseCode=PS
  M1: Turbine & Regulators : Subsystem
  M2 900 MVA : spsSynchronousMachinepuStandardLib/Synchronous Machine pu Standard  PresetModel=No  MechanicalLoad=Mechanical power Pm  ShowDetailedParameters=on  RotorType=Round  Units=per unit standard parameters  MeasurementBus=off  NominalParameters="[900E6  20000   60 ]"  Reactances1=[1.8 .3 .25 1.7 .55 .25 .2]  Reactances2=[ 1.305, 0.296, 0.252, 0.474, 0.243, 0.18 ]  dAxisTimeConstants=Open-circuit  qAxisTimeConstants=Open-circuit  TimeConstants1=[]  TimeConstants2=[8 .03 .4 .05]  TimeConstants3=[]  TimeConstants4=[]  TimeConstants5=[ 1.01, 0.053, 0.1 ]  TimeConstants6=[]  TimeConstants7=[]  TimeConstants8=[]  StatorResistance=0.0025  Mechanical="[ 6.5 0  4]"  PolePairs=4  InitialConditions=[0 -42.8075 0.788608 0.788608 0.788608 -9.54571 -129.546 110.454 1.86756]  SetSaturation=off  Saturation=[0.6404,0.7127,0.8441,0.9214,0.9956,1.082,1.19,1.316,1.457;0.7,0.7698,0.8872,0.9466,0.9969,1.046,1.1,1.151,1.201]  LoadFlowParameters=[2 700000000 0 0 0]  TsPowergui=0  TsBlock=-1  IterativeModel=Trapezoidal non iterative  IterativeDiscreteModel=Trapezoidal non iterative  BusType=swing  Pref=0  Qref=0  Qmin=-inf  Qmax=inf  PLF=0  QLF=0
      settings: SourceProductBaseCode=PS
  M2: Turbine & Regulators : Subsystem
  Pref 1 : Constant  Value=0.777778
  Pref 2 : Constant  Value=0.777689
  Snubber 1 : spsThreePhaseSeriesRLCLoadLib/Three-Phase Series RLC Load  LConnTagsString=A|B|C  Configuration=Y (grounded)  NominalVoltage=20000  Vabc=[1e3 1e3 1e3]  Vabcp=[1e3 1e3 1e3]  NominalFrequency=60  UnbalancedPower=off  ActivePower=1e6  InductivePower=0  CapacitivePower=1e7  Pabc=[10e3 9e3 11e3]  QLabc=[100 90 110]  QCabc=[100 90 110]  Pabcp=[10e3 9e3 11e3]  QLabcp=[100 90 110]  QCabcp=[100 90 110]  Measurements=None  LoadType=constant Z
  Snubber 2 : spsThreePhaseSeriesRLCLoadLib/Three-Phase Series RLC Load  LConnTagsString=A|B|C  Configuration=Y (grounded)  NominalVoltage=20000  Vabc=[1e3 1e3 1e3]  Vabcp=[1e3 1e3 1e3]  NominalFrequency=60  UnbalancedPower=off  ActivePower=1e6  InductivePower=0  CapacitivePower=1e7  Pabc=[10e3 9e3 11e3]  QLabc=[100 90 110]  QCabc=[100 90 110]  Pabcp=[10e3 9e3 11e3]  QLabcp=[100 90 110]  QCabcp=[100 90 110]  Measurements=None  LoadType=constant Z
  Stair Generator : spsStairGeneratorLib/Stair Generator  t=[0 15 20]  e=[0 1 0 ]  Ts=0
  Switch1 : Switch  Threshold=1  InputSameDT=on
  T1: 900MVA 20 kV-230 kV : spsThreePhaseTransformerTwoWindingsLib/Three-Phase Transformer (Two Windings)  Winding1Connection=Delta (D1)  Winding2Connection=Yg  CoreType=Three single-phase transformers  SetSaturation=off  Hysteresis=off  DataFile='hysteresis'  SetInitialFlux=off  Measurements=None  UNITS=pu  NominalPower="[ 900e6   60 ]"  Winding1="[ 20e3  1e-6   0  ]"  Winding2="[ 230e3  1e-6   0.15 ]"  Rm=500  Lm=500  L0=0.5  Saturation="[ 0,0  ;  0.005,1.2  ;  1.0,1.4 ]"  InitialFluxes=[ 0.8 , -0.8 , 0.7 ]  BreakLoop=off  DiscreteSolver=Trapezoidal iterative  DataType=off  TransfoNumber=0
  T2: 900MVA 20 kV/230 kV : spsThreePhaseTransformerTwoWindingsLib/Three-Phase Transformer (Two Windings)  Winding1Connection=Delta (D1)  Winding2Connection=Yg  CoreType=Three single-phase transformers  SetSaturation=off  Hysteresis=off  DataFile='hysteresis'  SetInitialFlux=off  Measurements=None  UNITS=pu  NominalPower=[ 900e6 60 ]  Winding1="[ 20e3 1e-6  0.0]"  Winding2=[ 230e3 1e-6 0.15]  Rm=500  Lm=500  L0=0.5  Saturation="[ 0,0  ;  0.005,1.2  ;  1.0,1.4 ]"  InitialFluxes=[ 0.8 , -0.8 , 0.7 ]  BreakLoop=off  DiscreteSolver=Trapezoidal iterative  DataType=off  TransfoNumber=0
  Vref1 : Constant
  Vref1 1 : Constant  Value=0.777689+0.05
  Vref2 : Constant
  Vref3 : Constant  Value=PSSMODEL
  Vref4 : Constant  Value=PSSMODEL
  sig : Subsystem
  sig1 : Subsystem
  " A" : PMIOPort  Side=Right
  " B" : PMIOPort  Port=2  Side=Right
  " C" : PMIOPort  Port=3  Side=Right
  wires:
  Pref 1/1 -> M1: Turbine & Regulators/2(Pref)
  Vref2/1 -> M2: Turbine & Regulators/3(Vref)
  Vref4/1 -> M2: Turbine & Regulators/4(PSS)
  sig/1(Out1) -> M1: Turbine & Regulators/1(m)
  M1 900 MVA/1 -> [m1]
  M2 900 MVA/1 -> [m2]
  [m1] -> sig/1(In1)
  Vref3/1 -> M1: Turbine & Regulators/4(PSS)
  sig1/1(Out1) -> M2: Turbine & Regulators/1(m)
  [m2] -> sig1/1(In1)
  Stair Generator/1 -> Switch1/2
  Pref 2/1 -> Switch1/3
  Vref1 1/1 -> Switch1/1
  Switch1/1 -> M2: Turbine & Regulators/2(Pref)
  Vref1/1 -> M1: Turbine & Regulators/3(Vref)
  M1: Turbine & Regulators/1(Pm) -> M1 900 MVA/1
  M1: Turbine & Regulators/2(Vf) -> M1 900 MVA/2
  M2: Turbine & Regulators/2(Vf) -> M2 900 MVA/2
  M2: Turbine & Regulators/1(Pm) -> M2 900 MVA/1
  connections:
  T1: 900MVA 20 kV-230 kV/RConn1 -- 25km Area 1/LConn1
  T1: 900MVA 20 kV-230 kV/RConn2 -- 25km Area 1/LConn2
  Snubber 2/LConn1 -- T2: 900MVA 20 kV/230 kV/LConn1 -- BG2/RConn1 -- Load Flow Bus1/LConn1
  Snubber 2/LConn2 -- T2: 900MVA 20 kV/230 kV/LConn2 -- BG2/RConn2
  Snubber 2/LConn3 -- BG2/RConn3 -- T2: 900MVA 20 kV/230 kV/LConn3
  T1: 900MVA 20 kV-230 kV/RConn3 -- 25km Area 1/LConn3
  10 km Area 1/RConn1 -- " A"/RConn1 -- 967MW 100MVAR -187MVAR/LConn1 -- -200MVAR/LConn1
  10 km Area 1/RConn2 -- " B"/RConn1 -- 967MW 100MVAR -187MVAR/LConn2 -- -200MVAR/LConn2
  10 km Area 1/RConn3 -- " C"/RConn1 -- 967MW 100MVAR -187MVAR/LConn3 -- -200MVAR/LConn3
  Snubber 1/LConn1 -- Load Flow Bus/LConn1 -- T1: 900MVA 20 kV-230 kV/LConn1 -- BG1/RConn1
  T1: 900MVA 20 kV-230 kV/LConn2 -- Snubber 1/LConn2 -- BG1/RConn2
  T1: 900MVA 20 kV-230 kV/LConn3 -- Snubber 1/LConn3 -- BG1/RConn3
  25km Area 1/RConn2 -- 10 km Area 1/LConn2 -- T2: 900MVA 20 kV/230 kV/RConn2
  25km Area 1/RConn1 -- 10 km Area 1/LConn1 -- T2: 900MVA 20 kV/230 kV/RConn1
  25km Area 1/RConn3 -- 10 km Area 1/LConn3 -- T2: 900MVA 20 kV/230 kV/RConn3
  M1 900 MVA/RConn1 -- BG1/LConn1
  M1 900 MVA/RConn2 -- BG1/LConn2
  M1 900 MVA/RConn3 -- BG1/LConn3
  M2 900 MVA/RConn1 -- BG2/LConn1
  M2 900 MVA/RConn2 -- BG2/LConn2
  M2 900 MVA/RConn3 -- BG2/LConn3

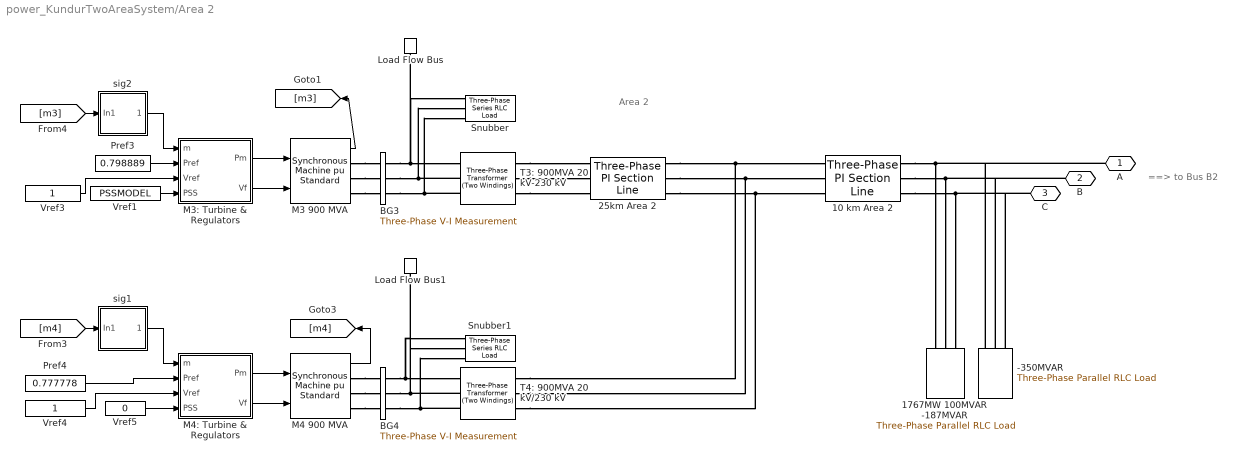
== system power_KundurTwoAreaSystem/Area 2 ==
  note: ==> to Bus B2
  note: Area 2
  -350MVAR : spsThreePhaseParallelRLCLoadLib/Three-Phase Parallel RLC Load  LConnTagsString=A|B|C  Configuration=Y (grounded)  NominalVoltage=230e3  Vabc=[1e3 1e3 1e3]  Vabcp=[1e3 1e3 1e3]  NominalFrequency=60  UnbalancedPower=off  ActivePower=0  InductivePower=0  CapacitivePower=350e6  Pabc=[10e3 9e3 11e3]  QLabc=[100 90 110]  QCabc=[100 90 110]  Pabcp=[10e3 9e3 11e3]  QLabcp=[100 90 110]  QCabcp=[100 90 110]  Measurements=None  LoadType=constant Z
  10 km Area 2 : spsThreePhasePISectionLineLib/Three-Phase PI Section Line  LConnTagsString=a|b|c  RConnTagsString=A|B|C  Length=10  Frequency=60  Resistances=[0.0001*529 1.61]  Inductances=[0.001*529/(377) 0.0061]  Capacitances=[0.00175/529/(377) 5.2489e-9]
  1767MW 100MVAR -187MVAR : spsThreePhaseParallelRLCLoadLib/Three-Phase Parallel RLC Load  LConnTagsString=A|B|C  Configuration=Y (grounded)  NominalVoltage=230e3  Vabc=[1e3 1e3 1e3]  Vabcp=[1e3 1e3 1e3]  NominalFrequency=60  UnbalancedPower=off  ActivePower=1767e6  InductivePower=100e6  CapacitivePower=187e6  Pabc=[10e3 9e3 11e3]  QLabc=[100 90 110]  QCabc=[100 90 110]  Pabcp=[10e3 9e3 11e3]  QLabcp=[100 90 110]  QCabcp=[100 90 110]  Measurements=None  LoadType=constant Z
  25km Area 2 : spsThreePhasePISectionLineLib/Three-Phase PI Section Line  LConnTagsString=a|b|c  RConnTagsString=A|B|C  Length=25  Frequency=60  Resistances=[0.0001*529 1.61]  Inductances=[0.001*529/(377) 0.0061]  Capacitances=[0.00175/529/(377) 5.2489e-9]
  BG3 : spsThreePhaseVIMeasurementLib/Three-Phase V-I Measurement  VoltageMeasurement=no  SetLabelV=on  LabelV=Vabc_G3  Vpu=on  VpuLL=off  CurrentMeasurement=no  SetLabelI=on  LabelI=Iabc_G3  Ipu=on  Pbase=900e6  Vbase=20e3  OutputType=Complex  PhasorSimulation=off  PSBequivalent=0
  BG4 : spsThreePhaseVIMeasurementLib/Three-Phase V-I Measurement  VoltageMeasurement=no  SetLabelV=on  LabelV=Vabc_G4  Vpu=on  VpuLL=off  CurrentMeasurement=no  SetLabelI=on  LabelI=Iabc_G4  Ipu=on  Pbase=900e6  Vbase=20e3  OutputType=Complex  PhasorSimulation=off  PSBequivalent=0
  Load Flow Bus : spsLoadFlowBusLib/Load Flow Bus  LConnTagsString=a  Phases=single  Connectors=on one side  ID=M3_Area2  Vbase=20e3  Vref=1  Vangle=0  VLF=1  VLFb=1  VLFc=1  angleLF=-16.02  angleLFb=0  angleLFc=0
      settings: AttributesFormatString=%<ID>\n%<Vbase>V\n%<VLF>pu\n%<angleLF>deg.  SourceProductBaseCode=PS
  Load Flow Bus1 : spsLoadFlowBusLib/Load Flow Bus  LConnTagsString=a  Phases=single  Connectors=on one side  ID=M4_Area2  Vbase=20e3  Vref=1  Vangle=0  VLF=1  VLFb=1  VLFc=1  angleLF=-26.66  angleLFb=0  angleLFc=0
      settings: AttributesFormatString=%<ID>\n%<Vbase>V\n%<VLF>pu\n%<angleLF>deg.  SourceProductBaseCode=PS
  M3 900 MVA : spsSynchronousMachinepuStandardLib/Synchronous Machine pu Standard  PresetModel=No  MechanicalLoad=Mechanical power Pm  ShowDetailedParameters=on  RotorType=Round  Units=per unit standard parameters  MeasurementBus=off  NominalParameters="[900E6  20000   60 ]"  Reactances1=[1.8 .3 .25 1.7 .55 .25 .2]  Reactances2=[ 1.305, 0.296, 0.252, 0.474, 0.243, 0.18 ]  dAxisTimeConstants=Open-circuit  qAxisTimeConstants=Open-circuit  TimeConstants1=[]  TimeConstants2=[8 .03 .4 .05]  TimeConstants3=[]  TimeConstants4=[]  TimeConstants5=[ 1.01, 0.053, 0.1 ]  TimeConstants6=[]  TimeConstants7=[]  TimeConstants8=[]  StatorResistance=0.0025  Mechanical="[ 6.175 0  4]"  PolePairs=4  InitialConditions=[0 -56.3243 0.8041 0.8041 0.8041 -22.4087 -142.409 97.5913 1.85092]  SetSaturation=off  Saturation=[0.6404,0.7127,0.8441,0.9214,0.9956,1.082,1.19,1.316,1.457;0.7,0.7698,0.8872,0.9466,0.9969,1.046,1.1,1.151,1.201]  LoadFlowParameters=[1 719000000 0 0 0]  TsPowergui=0  TsBlock=-1  IterativeModel=Trapezoidal non iterative  IterativeDiscreteModel=Trapezoidal non iterative  BusType=PV  Pref=719000000  Qref=0  Qmin=-inf  Qmax=inf  PLF=0  QLF=0
      settings: SourceProductBaseCode=PS
  M3: Turbine & Regulators : Subsystem
  M4 900 MVA : spsSynchronousMachinepuStandardLib/Synchronous Machine pu Standard  PresetModel=No  MechanicalLoad=Mechanical power Pm  ShowDetailedParameters=on  RotorType=Round  Units=per unit standard parameters  MeasurementBus=off  NominalParameters="[900E6  20000   60 ]"  Reactances1=[1.8 .3 .25 1.7 .55 .25 .2]  Reactances2=[ 1.305, 0.296, 0.252, 0.474, 0.243, 0.18 ]  dAxisTimeConstants=Open-circuit  qAxisTimeConstants=Open-circuit  TimeConstants1=[]  TimeConstants2=[8 .03 .4 .05]  TimeConstants3=[]  TimeConstants4=[]  TimeConstants5=[ 1.01, 0.053, 0.1 ]  TimeConstants6=[]  TimeConstants7=[]  TimeConstants8=[]  StatorResistance=0.0025  Mechanical="[ 6.175 0  4]"  PolePairs=4  InitialConditions=[0 -67.7513 0.783185 0.783185 0.783185 -33.268 -153.268 86.732 1.82209]  SetSaturation=off  Saturation=[0.6404,0.7127,0.8441,0.9214,0.9956,1.082,1.19,1.316,1.457;0.7,0.7698,0.8872,0.9466,0.9969,1.046,1.1,1.151,1.201]  LoadFlowParameters=[1 700000000 0 0 0]  TsPowergui=0  TsBlock=-1  IterativeModel=Trapezoidal non iterative  IterativeDiscreteModel=Trapezoidal non iterative  BusType=PV  Pref=700000000  Qref=0  Qmin=-inf  Qmax=inf  PLF=0  QLF=0
      settings: SourceProductBaseCode=PS
  M4: Turbine & Regulators : Subsystem
  Pref3 : Constant  Value=0.798889
  Pref4 : Constant  Value=0.777778
  Snubber : spsThreePhaseSeriesRLCLoadLib/Three-Phase Series RLC Load  LConnTagsString=A|B|C  Configuration=Y (grounded)  NominalVoltage=20000  Vabc=[1e3 1e3 1e3]  Vabcp=[1e3 1e3 1e3]  NominalFrequency=60  UnbalancedPower=off  ActivePower=1e6  InductivePower=0  CapacitivePower=1e7  Pabc=[10e3 9e3 11e3]  QLabc=[100 90 110]  QCabc=[100 90 110]  Pabcp=[10e3 9e3 11e3]  QLabcp=[100 90 110]  QCabcp=[100 90 110]  Measurements=None  LoadType=constant Z
  Snubber1 : spsThreePhaseSeriesRLCLoadLib/Three-Phase Series RLC Load  LConnTagsString=A|B|C  Configuration=Y (grounded)  NominalVoltage=20000  Vabc=[1e3 1e3 1e3]  Vabcp=[1e3 1e3 1e3]  NominalFrequency=60  UnbalancedPower=off  ActivePower=1e6  InductivePower=0  CapacitivePower=1e7  Pabc=[10e3 9e3 11e3]  QLabc=[100 90 110]  QCabc=[100 90 110]  Pabcp=[10e3 9e3 11e3]  QLabcp=[100 90 110]  QCabcp=[100 90 110]  Measurements=None  LoadType=constant Z
  T3: 900MVA 20 kV-230 kV : spsThreePhaseTransformerTwoWindingsLib/Three-Phase Transformer (Two Windings)  Winding1Connection=Delta (D1)  Winding2Connection=Yg  CoreType=Three single-phase transformers  SetSaturation=off  Hysteresis=off  DataFile='hysteresis'  SetInitialFlux=off  Measurements=None  UNITS=pu  NominalPower="[ 900e6   60 ]"  Winding1="[ 20e3  1e-6   0  ]"  Winding2="[ 230e3  1e-6   0.15 ]"  Rm=500  Lm=500  L0=0.5  Saturation="[ 0,0  ;  0.005,1.2  ;  1.0,1.4 ]"  InitialFluxes=[ 0.8 , -0.8 , 0.7 ]  BreakLoop=off  DiscreteSolver=Trapezoidal iterative  DataType=off  TransfoNumber=0
  T4: 900MVA 20 kV/230 kV : spsThreePhaseTransformerTwoWindingsLib/Three-Phase Transformer (Two Windings)  Winding1Connection=Delta (D1)  Winding2Connection=Yg  CoreType=Three single-phase transformers  SetSaturation=off  Hysteresis=off  DataFile='hysteresis'  SetInitialFlux=off  Measurements=None  UNITS=pu  NominalPower=[ 900e6 60 ]  Winding1="[ 20e3 1e-6  0.0]"  Winding2=[ 230e3 1e-6 0.15]  Rm=500  Lm=500  L0=0.5  Saturation="[ 0,0  ;  0.005,1.2  ;  1.0,1.4 ]"  InitialFluxes=[ 0.8 , -0.8 , 0.7 ]  BreakLoop=off  DiscreteSolver=Trapezoidal iterative  DataType=off  TransfoNumber=0
  Vref1 : Constant  Value=PSSMODEL
  Vref3 : Constant
  Vref4 : Constant
  Vref5 : Constant  Value=0
  sig1 : Subsystem
  sig2 : Subsystem
  A : PMIOPort  Side=Left
  B : PMIOPort  Port=2  Side=Left
  C : PMIOPort  Port=3  Side=Left
  wires:
  Pref3/1 -> M3: Turbine & Regulators/2(Pref)
  Vref3/1 -> M3: Turbine & Regulators/3(Vref)
  Pref4/1 -> M4: Turbine & Regulators/2(Pref)
  Vref4/1 -> M4: Turbine & Regulators/3(Vref)
  Vref5/1 -> M4: Turbine & Regulators/4(PSS)
  M3 900 MVA/1 -> [m3]
  M4 900 MVA/1 -> [m4]
  sig2/1(Out1) -> M3: Turbine & Regulators/1(m)
  sig1/1(Out1) -> M4: Turbine & Regulators/1(m)
  [m4] -> sig1/1(In1)
  [m3] -> sig2/1(In1)
  Vref1/1 -> M3: Turbine & Regulators/4(PSS)
  M3: Turbine & Regulators/1(Pm) -> M3 900 MVA/1
  M3: Turbine & Regulators/2(Vf) -> M3 900 MVA/2
  M4: Turbine & Regulators/1(Pm) -> M4 900 MVA/1
  M4: Turbine & Regulators/2(Vf) -> M4 900 MVA/2
  connections:
  T3: 900MVA 20 kV-230 kV/LConn3 -- BG3/RConn3 -- Snubber/LConn3
  T3: 900MVA 20 kV-230 kV/LConn2 -- BG3/RConn2 -- Snubber/LConn2
  Snubber/LConn1 -- Load Flow Bus/LConn1 -- T3: 900MVA 20 kV-230 kV/LConn1 -- BG3/RConn1
  T3: 900MVA 20 kV-230 kV/RConn3 -- 25km Area 2/LConn3
  T4: 900MVA 20 kV/230 kV/LConn3 -- Snubber1/LConn3 -- BG4/RConn3
  T4: 900MVA 20 kV/230 kV/LConn2 -- Snubber1/LConn2 -- BG4/RConn2
  Snubber1/LConn1 -- Load Flow Bus1/LConn1 -- BG4/RConn1 -- T4: 900MVA 20 kV/230 kV/LConn1
  T3: 900MVA 20 kV-230 kV/RConn2 -- 25km Area 2/LConn2
  T3: 900MVA 20 kV-230 kV/RConn1 -- 25km Area 2/LConn1
  25km Area 2/RConn2 -- 10 km Area 2/LConn2 -- T4: 900MVA 20 kV/230 kV/RConn2
  25km Area 2/RConn1 -- 10 km Area 2/LConn1 -- T4: 900MVA 20 kV/230 kV/RConn1
  25km Area 2/RConn3 -- 10 km Area 2/LConn3 -- T4: 900MVA 20 kV/230 kV/RConn3
  M3 900 MVA/RConn1 -- BG3/LConn1
  M3 900 MVA/RConn2 -- BG3/LConn2
  M3 900 MVA/RConn3 -- BG3/LConn3
  M4 900 MVA/RConn1 -- BG4/LConn1
  M4 900 MVA/RConn2 -- BG4/LConn2
  M4 900 MVA/RConn3 -- BG4/LConn3
  10 km Area 2/RConn1 -- A/RConn1 -- -350MVAR/LConn1 -- 1767MW 100MVAR -187MVAR/LConn1
  10 km Area 2/RConn2 -- 1767MW 100MVAR -187MVAR/LConn2 -- -350MVAR/LConn2 -- B/RConn1
  10 km Area 2/RConn3 -- -350MVAR/LConn3 -- C/RConn1 -- 1767MW 100MVAR -187MVAR/LConn3
